simulink model "linear_2_tank_model"  (R2019b)
settings: Solver=VariableStepAuto  StartTime=0.0  StopTime=10.0  RelTol=1e-3
values from neighbouring files (symbols this model uses):
  Ju = [[(gamma_1/(2*sqrt(beta_1+gamma_1*ue1))), 0];[0, 0]]    [script_task_2_linear.m]
  Jx = [[(-k_1/(2*sqrt(xe1))), 0]; [(k_1/(2*sqrt(xe1))), (-k_2/(2*sqrt(xe2)))]]    [script_task_2_linear.m]
  xe1 = (k_2*sqrt(xe2)/k_1)^2    [script_check_equilibrium.m]    (also in script_task_2_linear.m; script_task_2_nonlinear.m)
  xe2 = 25.53    [script_check_equilibrium.m]    (also in script_task_2_linear.m; script_task_2_nonlinear.m)
settings Model: Creator=NicSch02  LastModifiedBy=NicSch02

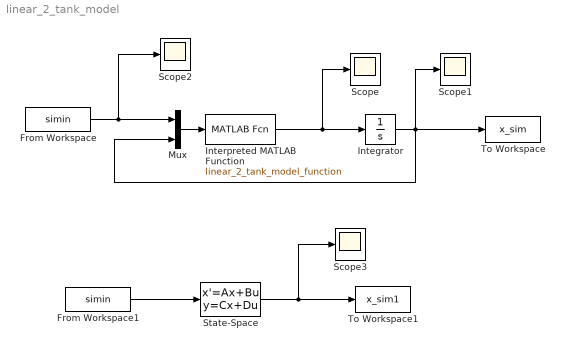
== system linear_2_tank_model ==
  From Workspace : FromWorkspace  VariableName=simin  SampleTime=0
  From Workspace1 : FromWorkspace  VariableName=simin  SampleTime=0
  Integrator : Integrator  InitialCondition=[xe1; xe2;]
  Interpreted MATLAB Function : MATLABFcn  MATLABFcn=linear_2_tank_model_function
  Mux : Mux  Inputs=2
  Scope{,1..3} (4 alike) : Scope
  State-Space : StateSpace  A=Jx  B=Ju  C=[0,1]  D=[0,0]  InitialCondition=[xe1; xe2]
  To Workspace : ToWorkspace  VariableName=x_sim  SaveFormat=Structure With Time  SampleTime=-1
  To Workspace1 : ToWorkspace  VariableName=x_sim1  SaveFormat=Structure With Time  SampleTime=-1
  wires:
  Interpreted MATLAB Function/1 -> Scope/1, Integrator/1
  From Workspace/1 -> Scope2/1, Mux/1
  Integrator/1 -> Scope1/1, Mux/2, To Workspace/1
  Mux/1 -> Interpreted MATLAB Function/1
  From Workspace1/1 -> State-Space/1
  State-Space/1 -> Scope3/1, To Workspace1/1
